simulink model "processor_with_peripherals"  (R2025a)
settings: Solver=FixedStepDiscrete  StartTime=0.0  StopTime=inf  RelTol=1e-3
libraries: simulink x6
(part 5 of 5)

== matlab function processor_with_peripherals/Processor/Core_0/Execute (EX) Stage/MATLAB Function ==
  data: Operand1 input; ALU_Result output int32 size=1; Operand2 input; ALUOp input; Instruction input; Zero_Flag output boolean size=1; AtomicOp input
function [ALU_Result, Zero_Flag] = alu(Operand1, Operand2, ALUOp, Instruction, AtomicOp)
% This is the final ALU code, supporting standard operations and
% the RISC-V "A" extension for atomic memory operations.

    instr = uint32(Instruction);
    alu_op_val = ALUOp(1)*2 + ALUOp(2); 

    % Extract function fields
    funct3 = bitshift(bitand(instr, uint32(hex2dec('7000'))), -12);
    funct7 = bitshift(bitand(instr, uint32(hex2dec('FE000000'))), -25);
    funct5 = bitshift(bitand(instr, uint32(hex2dec('F8000000'))), -27); % For atomic ops

    ALU_Result = int32(0);

    if AtomicOp
        % --- This is an Atomic Operation ---
        switch funct5
            case 0,  ALU_Result = Operand1 + Operand2;  % AMOADD.W
            case 1,  ALU_Result = Operand2;            % AMOSWAP.W
            case 4,  ALU_Result = bitxor(Operand1, Operand2); % AMOXOR.W
            case 12, ALU_Result = bitand(Operand1, Operand2); % AMOAND.W
            case 20, ALU_Result = bitor(Operand1, Operand2);  % AMOOR.W
            otherwise, ALU_Result = Operand1;
        end
    else
        % --- This is a Normal Operation ---
        switch alu_op_val
            case 0 % For LW, SW, ADDI, JAL, etc.
                ALU_Result = Operand1 + Operand2;
            case 1 % For Branches
                ALU_Result = Operand1 - Operand2;
            case 2 % R-type instructions
                switch funct3
                    case 0 % ADD or SUB
                        if funct7 == 32, ALU_Result = Operand1 - Operand2; else, ALU_Result = Operand1 + Operand2; end
                    case 1, ALU_Result = int32(bitshift(uint32(Operand1), Operand2)); % SLL
                    case 2, if Operand1 < Operand2, ALU_Result = int32(1); else, ALU_Result = int32(0); end % SLT
                    case 4, ALU_Result = bitxor(Operand1, Operand2); % XOR
                    case 6, ALU_Result = bitor(Operand1, Operand2);  % OR
                    case 7, ALU_Result = bitand(Operand1, Operand2); % AND
                    otherwise, ALU_Result = int32(0);
                end
            case 3 % I-type instructions
                 switch funct3
                    case 0, ALU_Result = Operand1 + Operand2; % ADDI
                    case 2, if Operand1 < Operand2, ALU_Result = int32(1); else, ALU_Result = int32(0); end % SLTI
                    case 4, ALU_Result = bitxor(Operand1, Operand2); % XORI
                    case 6, ALU_Result = bitor(Operand1, Operand2);  % ORI
                    case 7, ALU_Result = bitand(Operand1, Operand2); % ANDI
                    otherwise, ALU_Result = int32(0);
                 end
        end
    end
    
    Zero_Flag = (ALU_Result == 0);
end

== matlab function processor_with_peripherals/Processor/Core_0/Instruction Decode(ID) Stage/MATLAB Function2 ==
  data: ReadAddr1 input; ReadData1 output int32; ReadAddr2 input; WriteAddr input; WriteData input; WriteEnable input; ReadData2 output int32
function [ReadData1, ReadData2] = register_file(ReadAddr1, ReadAddr2, WriteAddr, WriteData, WriteEnable)
% Implements a 32-register file for a RISC-V processor.
% x0 is hardwired to zero. Uses 1-based MATLAB indexing.

    persistent Registers;
    if isempty(Registers)
        Registers = zeros(32, 1, 'int32');
    end

    % 1. Handle the Write-Back from the WB stage first (synchronous write)
    if WriteEnable
        if WriteAddr > 0 % Do not write to register x0
            % MATLAB arrays are 1-based, so we add 1 to the 0-based RISC-V address
            Registers(WriteAddr + 1) = WriteData;
        end
    end

    % 2. Perform the Reads for the ID stage (combinational read)
    if ReadAddr1 == 0
        ReadData1 = int32(0);
    else
        ReadData1 = Registers(ReadAddr1 + 1);
    end

    if ReadAddr2 == 0
        ReadData2 = int32(0);
    else
        ReadData2 = Registers(ReadAddr2 + 1);
    end
end

== matlab function processor_with_peripherals/Processor/Core_1/Execute (EX) Stage/MATLAB Function ==
  data: Operand1 input; ALU_Result output int32 size=1; Operand2 input; ALUOp input; Instruction input; Zero_Flag output boolean size=1; AtomicOp input
function [ALU_Result, Zero_Flag] = alu(Operand1, Operand2, ALUOp, Instruction, AtomicOp)
% This is the final ALU code, supporting standard operations and
% the RISC-V "A" extension for atomic memory operations.

    instr = uint32(Instruction);
    alu_op_val = ALUOp(1)*2 + ALUOp(2); 

    % Extract function fields
    funct3 = bitshift(bitand(instr, uint32(hex2dec('7000'))), -12);
    funct7 = bitshift(bitand(instr, uint32(hex2dec('FE000000'))), -25);
    funct5 = bitshift(bitand(instr, uint32(hex2dec('F8000000'))), -27); % For atomic ops

    ALU_Result = int32(0);

    if AtomicOp
        % --- This is an Atomic Operation ---
        switch funct5
            case 0,  ALU_Result = Operand1 + Operand2;  % AMOADD.W
            case 1,  ALU_Result = Operand2;            % AMOSWAP.W
            case 4,  ALU_Result = bitxor(Operand1, Operand2); % AMOXOR.W
            case 12, ALU_Result = bitand(Operand1, Operand2); % AMOAND.W
            case 20, ALU_Result = bitor(Operand1, Operand2);  % AMOOR.W
            otherwise, ALU_Result = Operand1;
        end
    else
        % --- This is a Normal Operation ---
        switch alu_op_val
            case 0 % For LW, SW, ADDI, JAL, etc.
                ALU_Result = Operand1 + Operand2;
            case 1 % For Branches
                ALU_Result = Operand1 - Operand2;
            case 2 % R-type instructions
                switch funct3
                    case 0 % ADD or SUB
                        if funct7 == 32, ALU_Result = Operand1 - Operand2; else, ALU_Result = Operand1 + Operand2; end
                    case 1, ALU_Result = int32(bitshift(uint32(Operand1), Operand2)); % SLL
                    case 2, if Operand1 < Operand2, ALU_Result = int32(1); else, ALU_Result = int32(0); end % SLT
                    case 4, ALU_Result = bitxor(Operand1, Operand2); % XOR
                    case 6, ALU_Result = bitor(Operand1, Operand2);  % OR
                    case 7, ALU_Result = bitand(Operand1, Operand2); % AND
                    otherwise, ALU_Result = int32(0);
                end
            case 3 % I-type instructions
                 switch funct3
                    case 0, ALU_Result = Operand1 + Operand2; % ADDI
                    case 2, if Operand1 < Operand2, ALU_Result = int32(1); else, ALU_Result = int32(0); end % SLTI
                    case 4, ALU_Result = bitxor(Operand1, Operand2); % XORI
                    case 6, ALU_Result = bitor(Operand1, Operand2);  % ORI
                    case 7, ALU_Result = bitand(Operand1, Operand2); % ANDI
                    otherwise, ALU_Result = int32(0);
                 end
        end
    end
    
    Zero_Flag = (ALU_Result == 0);
end

== matlab function processor_with_peripherals/Processor/Core_0/Instruction Fetch (IF) Stage/MATLAB Function ==
  data: vector_in input; scalar_out output uint32
function scalar_out = to_scalar(vector_in)
% This function extracts the first element from an input vector
% and ensures the output is a uint32 scalar.
    scalar_out = uint32(vector_in(1));
end

== matlab function processor_with_peripherals/Processor/Core_0/Instruction Decode(ID) Stage/MATLAB Function3 ==
  data: instruction input; rs1 output uint8; rs2 output uint8; rd output uint8
function [rs1, rs2, rd] = bit_slicer(instruction)
% This function correctly extracts the rs1, rs2, and rd fields
% from a 32-bit RISC-V instruction word.

    instr = uint32(instruction);

    % Extract rd (destination register, bits 11:7)
    rd  = uint8(bitshift(bitand(instr, uint32(hex2dec('F80'))), -7));

    % Extract rs1 (source register 1, bits 19:15)
    rs1 = uint8(bitshift(bitand(instr, uint32(hex2dec('F8000'))), -15));

    % Extract rs2 (source register 2, bits 24:20)
    rs2 = uint8(bitshift(bitand(instr, uint32(hex2dec('1F00000'))), -20));
end
